simulink model "RF_Receiver"  (R2022a)
settings: Solver=VariableStepAuto  StartTime=0.0  StopTime=10.0  RelTol=1e-3
values from neighbouring files (symbols this model uses):
  N = 3    [RFReceiverModelingForLteReceptionExample.m]
undefined symbols (not defined in the file or in its folder): magnitude, physconst, S
libraries: simrfV2util1 x4, dspstat3 x4, simrfV2elements x3, simulink_extras x2, dspmathops x2, simrfV2systems x1, commrflib2 x1, simrfV2sources1 x1
settings Model: Creator=The MathWorks, Inc.  LastModifiedBy=The MathWorks, Inc.
settings SolverCC: MaxZcPerStep=1
settings DataIOCC: ExternalInput=externalInput_tp3057db3b_3942_4699_a9d8_1b4b84f1b925  InitialState=initialState_tp3057db3b_3942_4699_a9d8_1b4b84f1b925  LoadExternalInput=on  LoadInitialState=on  SaveFinalState=on  SaveOperatingPoint=on  SaveFormat=Structure
settings DebuggingCC: UnconnectedInputMsg=warning  UnconnectedOutputMsg=warning  UnconnectedLineMsg=warning
settings RTWCC: DLArmComputeVersion=19.05

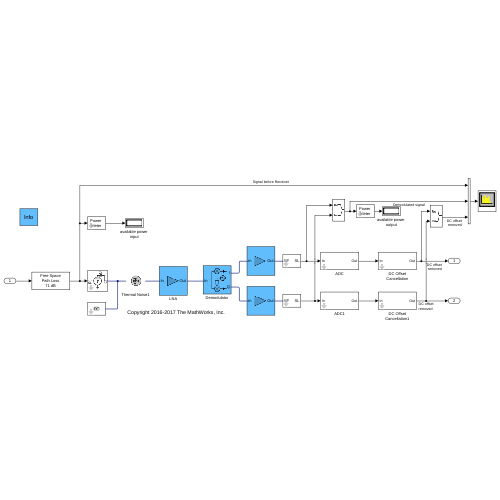
[thumbnail: Simulink's stored preview of the top-level diagram]
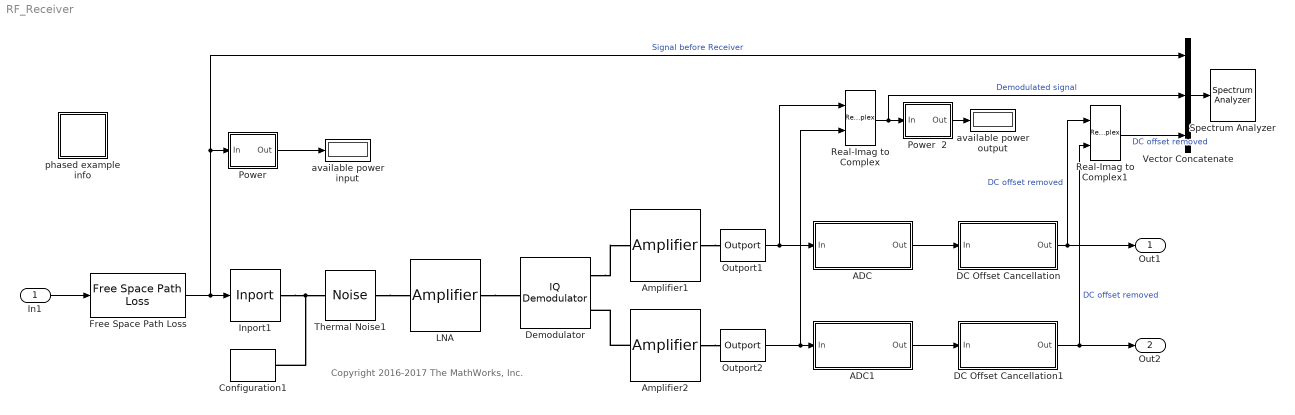
== system RF_Receiver ==
  note: Copyright 2016-2017 The MathWorks, Inc.
  In1 : Inport  PortDimensions=1  SampleTime=1.30208333333333e-07  Interpolate=off
      settings: SignalType=complex
  ADC : Subsystem  mask{Pmax=-30, N=10}
      mask prompts: Pmax "Full scale power (dBm)"; N "Number of bits"
  ADC1 : Subsystem  mask{Pmax=-30, N=10}
      mask prompts: Pmax "Full scale power (dBm)"; N "Number of bits"
  Amplifier1 : simrfV2elements/Amplifier  classname=amplifier  DataSource=Data file  File=unitygain.s2p  Paramtype=S-parameters  Sparam=[0 0;1 0]  SparamFreq=1e9 Hz  SparamZ0=50  Residues=0  Poles=0  DF={0 0; 1 0}  Source_linear_gain=Available power gain  linear_gain=15 dB  AmAmAmPmTable=[-25,5,-1;-10,20,-2;0,27,5;5,28,12]  Zin=50  Zout=50  Source_Poly=Odd order  Poly_Coeffs=[0 1]  IPType=Input  IP2=Inf dBm  IP3=11.3 dBm  P1dB=-2.5 dBm  Psat=inf dBm  Gcomp=inf dBm  InternalGrounding=on  SourceFreq=Extracted from data source  PlotFreq=[1e9:1e6:3e9] Hz  PlotType=X-Y plane  YParam1=S(1,1)  YFormat1=Magnitude (decibels)  YParam2=None  YFormat2=Magnitude (decibels)  YOption=Linear  XOption=Linear  SparamRepresentation=Time domain (rationalfit)  FitTol=-40  FitOpt=Fit individually  MaxPoles=48  AutoImpulseLength=on  ImpulseLength=1e-10 s  MagModeling=off  AddNoise=on  NoiseType=Noise figure  NoiseDist=White  NF=8.3  MinNF=0  Gopt=0  RN=0  CarrierFreq=0 Hz  NoiseAutoImpulseLength=on  NoiseImpulseLength=1e-10 s  ConstS21NL=on  OpFreq=0 Hz  SetOpFreqAsMaxS21=on
      settings: SourceProductBaseCode=RB
  Amplifier2 : simrfV2elements/Amplifier  classname=amplifier  DataSource=Data file  File=unitygain.s2p  Paramtype=S-parameters  Sparam=[0 0;1 0]  SparamFreq=1e9 Hz  SparamZ0=50  Residues=0  Poles=0  DF={0 0; 1 0}  Source_linear_gain=Available power gain  linear_gain=15 dB  AmAmAmPmTable=[-25,5,-1;-10,20,-2;0,27,5;5,28,12]  Zin=50  Zout=50  Source_Poly=Odd order  Poly_Coeffs=[0 1]  IPType=Input  IP2=Inf dBm  IP3=11.3 dBm  P1dB=-2.5 dBm  Psat=inf dBm  Gcomp=inf dBm  InternalGrounding=on  SourceFreq=Extracted from data source  PlotFreq=[1e9:1e6:3e9] Hz  PlotType=X-Y plane  YParam1=S(1,1)  YFormat1=Magnitude (decibels)  YParam2=None  YFormat2=Magnitude (decibels)  YOption=Linear  XOption=Linear  SparamRepresentation=Time domain (rationalfit)  FitTol=-40  FitOpt=Fit individually  MaxPoles=48  AutoImpulseLength=on  ImpulseLength=1e-10 s  MagModeling=off  AddNoise=on  NoiseType=Noise figure  NoiseDist=White  NF=8.3  MinNF=0  Gopt=0  RN=0  CarrierFreq=0 Hz  NoiseAutoImpulseLength=on  NoiseImpulseLength=1e-10 s  ConstS21NL=on  OpFreq=0 Hz  SetOpFreqAsMaxS21=on
      settings: SourceProductBaseCode=RB
  Configuration1 : simrfV2util1/Configuration  AutoFreq=off  Tones=[2.14] GHz  Harmonics=3  NormalizeCarrierPower=on  SolverType=Auto  UseCCode=on  StepSize=1.30208333333333e-07 s  AddNoise=on  defaultRNG=on  Seed=0  Temperature=290.0 K  SolverDelFlag=0  AbsTol=1e-6  RelTol=1e-3  MaxIter=10  ErrorEstimationType=2-norm over all variables  EnableInterpFilter=on  HiddenFIRfilterControllerParam=on  SmallSignalApprox=off  AllSimFreqs=on  SimFreqs=[] Hz  SimFreqsInternal=[]  SamplesPerFrame=1
      settings: SourceProductBaseCode=RB
  DC Offset Cancellation : Subsystem  mask(DC Offset Cancellation){N=32, V=N/2, ic=5e-4}
      mask prompts: N "Lenght of Averaging Filter (Samples):"; V "Buffer Overlap:"; ic "Initial Condition"
      mask help: Remove the DC offset by averaging the input signal.
      mask init:
      | V = N/2;
      mask Help:
      | Estimate the DC offeset of a signal using a running average filter, and removes it from the signal itself
      | This model uses components from the DSP System Toolbox.
      mask TypeOptions N: Buffer/N
      mask TypeOptions V: Buffer/V
      mask TypeOptions ic: Buffer/ic
  DC Offset Cancellation1 : Subsystem  mask(DC Offset Cancellation){N=32, V=N/2, ic=5e-4}
      mask prompts: N "Lenght of Averaging Filter (Samples):"; V "Buffer Overlap:"; ic "Initial Condition"
      mask help: Remove the DC offset by averaging the input signal.
      mask init:
      | V = N/2;
      mask Help:
      | Estimate the DC offeset of a signal using a running average filter, and removes it from the signal itself
      | This model uses components from the DSP System Toolbox.
      mask TypeOptions N: Buffer/N
      mask TypeOptions V: Buffer/V
      mask TypeOptions ic: Buffer/ic
  Demodulator : simrfV2systems/IQ Demodulator  classname=iqdemod  Source_linear_gain=Available power gain  linear_gain=2.3 dB  Poly_Coeffs=[0 1]  LOFreq=2.14 GHz  Zin=50  Zout=50  AddIRFilter=off  AddCSFilters=on  InternalGrounding=on  ForceNextInit=off  Source_Poly=Even and odd order  IPType=Input  IP2=56 dBm  IP3=25.9 dBm  P1dB=inf dBm  Psat=inf dBm  Gcomp=inf dBm  NF=10.9  GainMismatch=0.05 dB  PhaseMismatch=2 deg  Isolation=65 dB  AddPhaseNoise=on  PhaseNoiseOffset=[100e3 500e3 1e6]  PhaseNoiseLevel=[-110 -139 -145]  AutoImpulseLengthPN=on  ImpulseLengthPN=1e-10  ImpulseLength_unitPN=s  DesignMethodIR=Ideal  ResponseTypeIR=Highpass  ImplementationIR=LC Tee  ImplementationIdealIR=Constant per carrier  ImplementationRationalIR=Transfer function  UseFilterOrderIR=on  FilterOrderIR=3  PassFreq_lpIR=2.19  PassFreq_lp_unitIR=GHz  PassFreq_hpIR=2.09  PassFreq_hp_unitIR=GHz  PassFreq_bpIR=[2.09 2.19]  PassFreq_bp_unitIR=GHz  PassFreq_bsIR=[0 2.089999999]  PassFreq_bs_unitIR=GHz  PassAttenIR=10*log10(2)  StopFreq_lpIR=2.190000001  StopFreq_lp_unitIR=GHz  StopFreq_hpIR=2.089999999  StopFreq_hp_unitIR=GHz  StopFreq_bpIR=[2.089999999 2.190000001]  StopFreq_bp_unitIR=GHz  StopFreq_bsIR=[1e-09 2.09]  StopFreq_bs_unitIR=GHz  StopAttenIR=40  RsrcIR=50  RloadIR=50  AutoImpulseLengthIR=on  ImpulseLengthIR=1e-10  ImpulseLength_unitIR=s  DesignMethodCS=Ideal  ResponseTypeCS=Lowpass  ImplementationCS=LC Tee  ImplementationIdealCS=Constant per carrier  ImplementationRationalCS=Transfer function  UseFilterOrderCS=on  FilterOrderCS=3  PassFreq_lpCS=50  PassFreq_lp_unitCS=MHz  PassFreq_hpCS=0  PassFreq_hp_unitCS=Hz  PassFreq_bpCS=[0 50]  PassFreq_bp_unitCS=MHz  PassFreq_bsCS=[4.229999999 4.330000001]  PassFreq_bs_unitCS=GHz  PassAttenCS=10*log10(2)  StopFreq_lpCS=50.000001  StopFreq_lp_unitCS=MHz  StopFreq_hpCS=0  StopFreq_hp_unitCS=Hz  StopFreq_bpCS=[0 50.000001]  StopFreq_bp_unitCS=MHz  StopFreq_bsCS=[4.23 4.33]  StopFreq_bs_unitCS=GHz  StopAttenCS=40  RsrcCS=50  RloadCS=50  AutoImpulseLengthCS=on  ImpulseLengthCS=1e-10  ImpulseLength_unitCS=s
      settings: SourceProductBaseCode=RB
  Free Space Path Loss : commrflib2/Free Space Path Loss  mode=Decibels  dB=-10*log10(7.9433e-8)  d=0.100  fc=1920
      settings: SourceProductBaseCode=CM
  Inport1 : simrfV2util1/Inport  SimulinkInputSignalType=Power  CarrierFreq=[2.14] GHz  ZS=50  InternalGrounding=on
      settings: SourceProductBaseCode=RB
  LNA : simrfV2elements/Amplifier  classname=amplifier  DataSource=Data file  File=unitygain.s2p  Paramtype=S-parameters  Sparam=[0 0;1 0]  SparamFreq=1e9 Hz  SparamZ0=50  Residues=0  Poles=0  DF={0 0; 1 0}  Source_linear_gain=Available power gain  linear_gain=11.4 dB  AmAmAmPmTable=[-25,5,-1;-10,20,-2;0,27,5;5,28,12]  Zin=50  Zout=50  Source_Poly=Odd order  Poly_Coeffs=[0 1]  IPType=Input  IP2=Inf dBm  IP3=-6.6 dBm  P1dB=-12 dBm  Psat=inf dBm  Gcomp=inf dBm  InternalGrounding=on  SourceFreq=Extracted from data source  PlotFreq=[1e9:1e6:3e9] Hz  PlotType=X-Y plane  YParam1=S(1,1)  YFormat1=Magnitude (decibels)  YParam2=None  YFormat2=Magnitude (decibels)  YOption=Linear  XOption=Linear  SparamRepresentation=Time domain (rationalfit)  FitTol=-40  FitOpt=Fit individually  MaxPoles=48  AutoImpulseLength=on  ImpulseLength=1e-10 s  MagModeling=off  AddNoise=on  NoiseType=Noise figure  NoiseDist=White  NF=1.2  MinNF=0  Gopt=0  RN=0  CarrierFreq=0 Hz  NoiseAutoImpulseLength=on  NoiseImpulseLength=1e-10 s  ConstS21NL=on  OpFreq=0 Hz  SetOpFreqAsMaxS21=on
      settings: SourceProductBaseCode=RB
  Outport1 : simrfV2util1/Outport  SensorType=Power  OutputFormat=Real Passband  CarrierFreq=[0] Hz  ZL=50  InternalGrounding=on  StepSize=1e-6 s  AutoStep=on
      settings: SourceProductBaseCode=RB
  Outport2 : simrfV2util1/Outport  SensorType=Power  OutputFormat=Real Passband  CarrierFreq=[0] Hz  ZL=50  InternalGrounding=on  StepSize=1e-6 s  AutoStep=on
      settings: SourceProductBaseCode=RB
  "Power  " : Subsystem  mask{R=1}
      mask prompts: R "Reference Impedance [Ohm]"
      mask DialogControl DescGroupVar Prompt: Power Meter
      mask Display: disp('Power \nMeter')
  Power  2 : Subsystem  mask{R=1}
      mask prompts: R "Reference Impedance [Ohm]"
      mask DialogControl DescGroupVar Prompt: Power Meter
      mask Display: disp('Power \nMeter')
  Real-Imag to Complex : RealImagToComplex
  Real-Imag to Complex1 : RealImagToComplex
  Spectrum Analyzer : SpectrumAnalyzer
  Thermal Noise1 : simrfV2sources1/Noise  SimulinkInputSignalType=Ideal voltage  NoiseType=White  NoisePSD=4*physconst('Boltzmann')*290*50  CarrierFreq=0 Hz  AutoImpulseLength=on  ImpulseLength=1e-10 s  InternalGrounding=off
      settings: SourceProductBaseCode=RB
  Vector Concatenate : Concatenate  NumInputs=3  Mode=Multidimensional array  ConcatenateDimension=2
  available power input : Display
  available power output : Display
  phased example info : Subsystem
      settings: OpenFcn=showdemo('simrfV2_lte_receiver_script')
      mask Display: disp('Info')
  Out1 : Outport  PortDimensions=1  SampleTime=1.30208333333333e-07
  Out2 : Outport  Port=2  PortDimensions=1  SampleTime=1.30208333333333e-07
  wires:
  Outport1/1 -> Real-Imag to Complex/1, ADC/1(In)
  Outport2/1 -> Real-Imag to Complex/2, ADC1/1(In)
  In1/1 -> Free Space Path Loss/1
  ADC/1(Out) -> DC Offset Cancellation/1(In)
  ADC1/1(Out) -> DC Offset Cancellation1/1(In)
  DC Offset Cancellation/1(Out) -> Real-Imag to Complex1/1, Out1/1  "DC offset removed"
  DC Offset Cancellation1/1(Out) -> Real-Imag to Complex1/2, Out2/1  "DC offset removed"
  "Power  "/1(Out) -> available power input/1
  Power  2/1(Out) -> available power output/1
  Free Space Path Loss/1 -> Vector Concatenate/1, "Power  "/1(In), Inport1/1  "Signal before Receiver"
  Real-Imag to Complex/1 -> Vector Concatenate/2, Power  2/1(In)  "Demodulated signal"
  Real-Imag to Complex1/1 -> Vector Concatenate/3  "DC offset removed"
  Vector Concatenate/1 -> Spectrum Analyzer/1
  connections:
  Configuration1/LConn1 -- Inport1/RConn1 -- Thermal Noise1/RConn1
  Thermal Noise1/LConn1 -- LNA/LConn1
  LNA/RConn1 -- Demodulator/LConn1
  Demodulator/RConn1 -- Amplifier1/LConn1
  Amplifier2/LConn1 -- Demodulator/RConn2
  Amplifier1/RConn1 -- Outport1/LConn1
  Amplifier2/RConn1 -- Outport2/LConn1

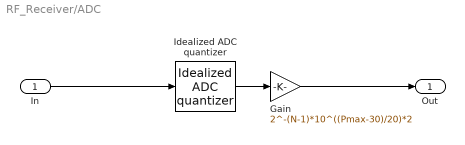
== system RF_Receiver/ADC ==
  In : Inport
  Gain : Gain  Gain=2^-(N-1)*10^((Pmax-30)/20)*2
  Idealized ADC quantizer : simulink_extras/Additional Discrete/Idealized ADC quantizer  NumberOfConverterBits=N  Vmin=-10^((Pmax-30)/20)*2  Vmax=10^((Pmax-30)/20)*2  OutputDataType=double  OutputNegativeValues=on
  Out : Outport  VectorParamsAs1DForOutWhenUnconnected=off
  wires:
  Gain/1 -> Out/1
  In/1 -> Idealized ADC quantizer/1
  Idealized ADC quantizer/1 -> Gain/1

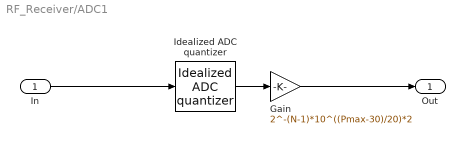
== system RF_Receiver/ADC1 ==
  In : Inport
  Gain : Gain  Gain=2^-(N-1)*10^((Pmax-30)/20)*2
  Idealized ADC quantizer : simulink_extras/Additional Discrete/Idealized ADC quantizer  NumberOfConverterBits=N  Vmin=-10^((Pmax-30)/20)*2  Vmax=10^((Pmax-30)/20)*2  OutputDataType=double  OutputNegativeValues=on
  Out : Outport  VectorParamsAs1DForOutWhenUnconnected=off
  wires:
  Idealized ADC quantizer/1 -> Gain/1
  In/1 -> Idealized ADC quantizer/1
  Gain/1 -> Out/1

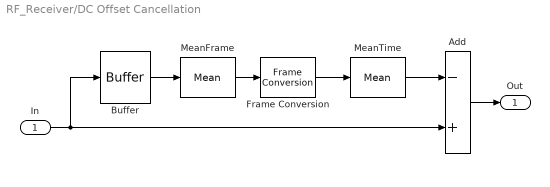
== system RF_Receiver/DC Offset Cancellation ==
  In : Inport
  Add : Sum  Inputs=-+
  Buffer : Buffer  N=N  V=V  ic=ic
  Frame Conversion : FrameConversion  OutFrame=Sample-based
  MeanFrame : dspstat3/Mean  run=on  InputProcessing=Columns as channels (frame based)  reset_popup=None  directionMode=Entire input  dimension=1  roiEnable=off  roiType=Rectangles  roiPortion=Entire ROI  roiOutput=Individual statistics for each ROI  roiFlag=off  roundingMode=Floor  overflowMode=off  outputDataTypeStr=Inherit: Same as accumulator  outputMin=[]  outputMax=[]  outputLastDataTypeStr=Inherit: Same as accumulator
  MeanTime : dspstat3/Mean  run=off  InputProcessing=Columns as channels (frame based)  reset_popup=None  directionMode=Entire input  dimension=1  roiEnable=off  roiType=Rectangles  roiPortion=Entire ROI  roiOutput=Individual statistics for each ROI  roiFlag=off  roundingMode=Floor  overflowMode=off  outputDataTypeStr=Inherit: Same as accumulator  outputMin=[]  outputMax=[]  outputLastDataTypeStr=Inherit: Same as accumulator
  Out : Outport  VectorParamsAs1DForOutWhenUnconnected=off
  wires:
  Buffer/1 -> MeanFrame/1
  In/1 -> Buffer/1, Add/2
  MeanFrame/1 -> Frame Conversion/1
  Add/1 -> Out/1
  MeanTime/1 -> Add/1
  Frame Conversion/1 -> MeanTime/1

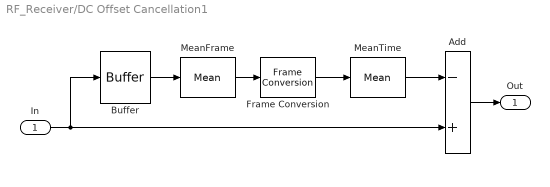
== system RF_Receiver/DC Offset Cancellation1 ==
  In : Inport
  Add : Sum  Inputs=-+
  Buffer : Buffer  N=N  V=V  ic=ic
  Frame Conversion : FrameConversion  OutFrame=Sample-based
  MeanFrame : dspstat3/Mean  run=on  InputProcessing=Columns as channels (frame based)  reset_popup=None  directionMode=Entire input  dimension=1  roiEnable=off  roiType=Rectangles  roiPortion=Entire ROI  roiOutput=Individual statistics for each ROI  roiFlag=off  roundingMode=Floor  overflowMode=off  outputDataTypeStr=Inherit: Same as accumulator  outputMin=[]  outputMax=[]  outputLastDataTypeStr=Inherit: Same as accumulator
  MeanTime : dspstat3/Mean  run=off  InputProcessing=Columns as channels (frame based)  reset_popup=None  directionMode=Entire input  dimension=1  roiEnable=off  roiType=Rectangles  roiPortion=Entire ROI  roiOutput=Individual statistics for each ROI  roiFlag=off  roundingMode=Floor  overflowMode=off  outputDataTypeStr=Inherit: Same as accumulator  outputMin=[]  outputMax=[]  outputLastDataTypeStr=Inherit: Same as accumulator
  Out : Outport  VectorParamsAs1DForOutWhenUnconnected=off
  wires:
  Frame Conversion/1 -> MeanTime/1
  MeanTime/1 -> Add/1
  Add/1 -> Out/1
  MeanFrame/1 -> Frame Conversion/1
  In/1 -> Add/2, Buffer/1
  Buffer/1 -> MeanFrame/1

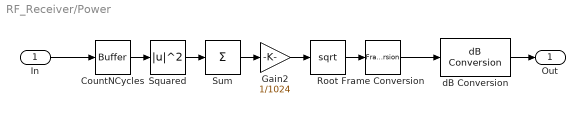
== system RF_Receiver/Power   ==
  In : Inport
  CountNCycles : Buffer  N=1024
  Frame Conversion : FrameConversion  OutFrame=Sample-based
  Gain2 : Gain  Gain=1/1024
  Root : Sqrt
  Squared : Math  Operator=magnitude^2  SignedPower=on
  Sum : Sum  Inputs=+
  dB Conversion : dspmathops/dB Conversion  dBtype=dBm  intype=Amplitude  R=R  fuzz=on
  Out : Outport  VectorParamsAs1DForOutWhenUnconnected=off
  wires:
  dB Conversion/1 -> Out/1
  In/1 -> CountNCycles/1
  Frame Conversion/1 -> dB Conversion/1
  CountNCycles/1 -> Squared/1
  Squared/1 -> Sum/1
  Sum/1 -> Gain2/1
  Root/1 -> Frame Conversion/1
  Gain2/1 -> Root/1

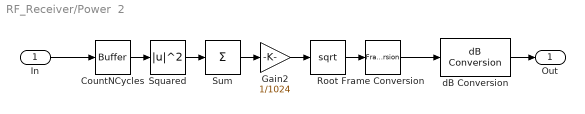
== system RF_Receiver/Power  2 ==
  In : Inport
  CountNCycles : Buffer  N=1024
  Frame Conversion : FrameConversion  OutFrame=Sample-based
  Gain2 : Gain  Gain=1/1024
  Root : Sqrt
  Squared : Math  Operator=magnitude^2  SignedPower=on
  Sum : Sum  Inputs=+
  dB Conversion : dspmathops/dB Conversion  dBtype=dBm  intype=Amplitude  R=R  fuzz=on
  Out : Outport  VectorParamsAs1DForOutWhenUnconnected=off
  wires:
  dB Conversion/1 -> Out/1
  In/1 -> CountNCycles/1
  Frame Conversion/1 -> dB Conversion/1
  CountNCycles/1 -> Squared/1
  Squared/1 -> Sum/1
  Sum/1 -> Gain2/1
  Root/1 -> Frame Conversion/1
  Gain2/1 -> Root/1

== system RF_Receiver/phased example info ==
